simulink model "DFADAS2_SenFus_v1_201204RC_training_210115"  (R2018b)
settings: Solver=FixedStepDiscrete  StartTime=0.0  StopTime=inf  FixedStep=0.002  RelTol=1e-3  EnableMultiTasking=on
PreLoadFcn:
  | RTWConfigurationCB('preloadfcn', bdroot);
libraries: canmsglib x108, simulink x48, canfdmsglib x12
(part 28 of 28)

== system DFADAS2_SenFus_v1_201204RC_training_210115/Signal Input (Input)/Signal Input (50ms) (Input50)/Cmr/CmrInfo/L1 Information (L1Info)/CAN Diagnosis (CANDia)/CheckSum Diagnosis (ChkSumDia)/Bit Check(BChk)/Bit Operating (BOp)/ChksumPre4 ==
  In1 : Inport
  Data Type Conversion8 : DataTypeConversion  OutDataTypeStr=uint16
  Extract Bits1 : simulink/Logic and Bit Operations/Extract Bits  bitsToExtract=Range of bits  numBits=8  bitIdxRange=4  outScalingMode=Treat bit field as an integer
      settings: SourceProductName=Simulink
  Out1 : Outport
  wires:
  Extract Bits1/1 -> Data Type Conversion8/1
  In1/1 -> Extract Bits1/1
  Data Type Conversion8/1 -> Out1/1

== system DFADAS2_SenFus_v1_201204RC_training_210115/Signal Input (Input)/Signal Input (50ms) (Input50)/Cmr/CmrInfo/L1 Information (L1Info)/CAN Diagnosis (CANDia)/CheckSum Diagnosis (ChkSumDia)/Bit Check(BChk)/Bit Operating (BOp)/ChksumPre5 ==
  In1 : Inport
  In2 : Inport  Port=2
  Add : Sum
  Data Type Conversion1 : DataTypeConversion  OutDataTypeStr=uint16
  Data Type Conversion4 : DataTypeConversion  OutDataTypeStr=uint16
  Shift Arithmetic2 : ArithShift  BitShiftNumber=-8
  Out1 : Outport
  wires:
  In1/1 -> Data Type Conversion4/1
  In2/1 -> Data Type Conversion1/1
  Shift Arithmetic2/1 -> Add/1
  Add/1 -> Out1/1
  Data Type Conversion4/1 -> Shift Arithmetic2/1
  Data Type Conversion1/1 -> Add/2

== system DFADAS2_SenFus_v1_201204RC_training_210115/Signal Input (Input)/Signal Input (50ms) (Input50)/Cmr/CmrInfo/L1 Information (L1Info)/CAN Diagnosis (CANDia)/CheckSum Diagnosis (ChkSumDia)/Bit Check(BChk)/Bit Operating (BOp)/ChksumPre6 ==
  In1 : Inport
  In2 : Inport  Port=2
  Add : Sum
  Data Type Conversion1 : DataTypeConversion  OutDataTypeStr=uint16
  Data Type Conversion4 : DataTypeConversion  OutDataTypeStr=uint16
  Shift Arithmetic2 : ArithShift  BitShiftNumber=-8
  Out1 : Outport
  wires:
  Data Type Conversion1/1 -> Add/2
  Data Type Conversion4/1 -> Shift Arithmetic2/1
  Add/1 -> Out1/1
  Shift Arithmetic2/1 -> Add/1
  In2/1 -> Data Type Conversion1/1
  In1/1 -> Data Type Conversion4/1

== system DFADAS2_SenFus_v1_201204RC_training_210115/Signal Input (Input)/Signal Input (50ms) (Input50)/Cmr/CmrInfo/L1 Information (L1Info)/CAN Diagnosis (CANDia)/CheckSum Diagnosis (ChkSumDia)/Bit Check(BChk)/Bit Operating (BOp)/ChksumPre7 ==
  In1 : Inport
  Data Type Conversion8 : DataTypeConversion  OutDataTypeStr=uint16
  Extract Bits1 : simulink/Logic and Bit Operations/Extract Bits  bitsToExtract=Range of bits  numBits=8  bitIdxRange=7  outScalingMode=Treat bit field as an integer
      settings: SourceProductName=Simulink
  Out1 : Outport
  wires:
  Data Type Conversion8/1 -> Out1/1
  In1/1 -> Extract Bits1/1
  Extract Bits1/1 -> Data Type Conversion8/1

== system DFADAS2_SenFus_v1_201204RC_training_210115/Signal Input (Input)/Signal Input (50ms) (Input50)/Cmr/CmrInfo/R0 Information (R0Info)/CAN Diagnosis (CANDia)/CheckSum Diagnosis (ChkSumDia)/Bit Check(BChk)/Bit Operating (BOp)/ChksumPre1 ==
  In1 : Inport
  Data Type Conversion7 : DataTypeConversion  OutDataTypeStr=uint16
  Out1 : Outport
  wires:
  In1/1 -> Data Type Conversion7/1
  Data Type Conversion7/1 -> Out1/1

== system DFADAS2_SenFus_v1_201204RC_training_210115/Signal Input (Input)/Signal Input (50ms) (Input50)/Cmr/CmrInfo/R0 Information (R0Info)/CAN Diagnosis (CANDia)/CheckSum Diagnosis (ChkSumDia)/Bit Check(BChk)/Bit Operating (BOp)/ChksumPre2 ==
  In1 : Inport
  Data Type Conversion7 : DataTypeConversion  OutDataTypeStr=uint16
  Extract Bits : simulink/Logic and Bit Operations/Extract Bits  bitsToExtract=Range of bits  numBits=8  bitIdxRange=6  outScalingMode=Treat bit field as an integer
      settings: SourceProductName=Simulink
  Out1 : Outport
  wires:
  Data Type Conversion7/1 -> Out1/1
  In1/1 -> Extract Bits/1
  Extract Bits/1 -> Data Type Conversion7/1

== system DFADAS2_SenFus_v1_201204RC_training_210115/Signal Input (Input)/Signal Input (50ms) (Input50)/Cmr/CmrInfo/R0 Information (R0Info)/CAN Diagnosis (CANDia)/CheckSum Diagnosis (ChkSumDia)/Bit Check(BChk)/Bit Operating (BOp)/ChksumPre3 ==
  In1 : Inport
  Data Type Conversion8 : DataTypeConversion  OutDataTypeStr=uint16
  Extract Bits1 : simulink/Logic and Bit Operations/Extract Bits  bitsToExtract=Range of bits  numBits=8  bitIdxRange=5  outScalingMode=Treat bit field as an integer
      settings: SourceProductName=Simulink
  Out1 : Outport
  wires:
  Data Type Conversion8/1 -> Out1/1
  In1/1 -> Extract Bits1/1
  Extract Bits1/1 -> Data Type Conversion8/1

== system DFADAS2_SenFus_v1_201204RC_training_210115/Signal Input (Input)/Signal Input (50ms) (Input50)/Cmr/CmrInfo/R0 Information (R0Info)/CAN Diagnosis (CANDia)/CheckSum Diagnosis (ChkSumDia)/Bit Check(BChk)/Bit Operating (BOp)/ChksumPre4 ==
  In1 : Inport
  Data Type Conversion8 : DataTypeConversion  OutDataTypeStr=uint16
  Extract Bits1 : simulink/Logic and Bit Operations/Extract Bits  bitsToExtract=Range of bits  numBits=8  bitIdxRange=4  outScalingMode=Treat bit field as an integer
      settings: SourceProductName=Simulink
  Out1 : Outport
  wires:
  Extract Bits1/1 -> Data Type Conversion8/1
  In1/1 -> Extract Bits1/1
  Data Type Conversion8/1 -> Out1/1

== system DFADAS2_SenFus_v1_201204RC_training_210115/Signal Input (Input)/Signal Input (50ms) (Input50)/Cmr/CmrInfo/R0 Information (R0Info)/CAN Diagnosis (CANDia)/CheckSum Diagnosis (ChkSumDia)/Bit Check(BChk)/Bit Operating (BOp)/ChksumPre5 ==
  In1 : Inport
  In2 : Inport  Port=2
  Add : Sum
  Data Type Conversion1 : DataTypeConversion  OutDataTypeStr=uint16
  Data Type Conversion4 : DataTypeConversion  OutDataTypeStr=uint16
  Shift Arithmetic2 : ArithShift  BitShiftNumber=-8
  Out1 : Outport
  wires:
  In1/1 -> Data Type Conversion4/1
  In2/1 -> Data Type Conversion1/1
  Shift Arithmetic2/1 -> Add/1
  Add/1 -> Out1/1
  Data Type Conversion4/1 -> Shift Arithmetic2/1
  Data Type Conversion1/1 -> Add/2

== system DFADAS2_SenFus_v1_201204RC_training_210115/Signal Input (Input)/Signal Input (50ms) (Input50)/Cmr/CmrInfo/R0 Information (R0Info)/CAN Diagnosis (CANDia)/CheckSum Diagnosis (ChkSumDia)/Bit Check(BChk)/Bit Operating (BOp)/ChksumPre6 ==
  In1 : Inport
  In2 : Inport  Port=2
  Add : Sum
  Data Type Conversion1 : DataTypeConversion  OutDataTypeStr=uint16
  Data Type Conversion4 : DataTypeConversion  OutDataTypeStr=uint16
  Shift Arithmetic2 : ArithShift  BitShiftNumber=-8
  Out1 : Outport
  wires:
  Data Type Conversion1/1 -> Add/2
  Data Type Conversion4/1 -> Shift Arithmetic2/1
  Add/1 -> Out1/1
  Shift Arithmetic2/1 -> Add/1
  In2/1 -> Data Type Conversion1/1
  In1/1 -> Data Type Conversion4/1

== system DFADAS2_SenFus_v1_201204RC_training_210115/Signal Input (Input)/Signal Input (50ms) (Input50)/Cmr/CmrInfo/R0 Information (R0Info)/CAN Diagnosis (CANDia)/CheckSum Diagnosis (ChkSumDia)/Bit Check(BChk)/Bit Operating (BOp)/ChksumPre7 ==
  In1 : Inport
  Data Type Conversion8 : DataTypeConversion  OutDataTypeStr=uint16
  Extract Bits1 : simulink/Logic and Bit Operations/Extract Bits  bitsToExtract=Range of bits  numBits=8  bitIdxRange=7  outScalingMode=Treat bit field as an integer
      settings: SourceProductName=Simulink
  Out1 : Outport
  wires:
  Data Type Conversion8/1 -> Out1/1
  In1/1 -> Extract Bits1/1
  Extract Bits1/1 -> Data Type Conversion8/1

== system DFADAS2_SenFus_v1_201204RC_training_210115/Signal Input (Input)/Signal Input (50ms) (Input50)/Cmr/CmrInfo/R1 Information (R1Info)/CAN Diagnosis (CANDia)/CheckSum Diagnosis (ChkSumDia)/Bit Check(BChk)/Bit Operating (BOp)/ChksumPre1 ==
  In1 : Inport
  Data Type Conversion7 : DataTypeConversion  OutDataTypeStr=uint16
  Out1 : Outport
  wires:
  Data Type Conversion7/1 -> Out1/1
  In1/1 -> Data Type Conversion7/1

== system DFADAS2_SenFus_v1_201204RC_training_210115/Signal Input (Input)/Signal Input (50ms) (Input50)/Cmr/CmrInfo/R1 Information (R1Info)/CAN Diagnosis (CANDia)/CheckSum Diagnosis (ChkSumDia)/Bit Check(BChk)/Bit Operating (BOp)/ChksumPre2 ==
  In1 : Inport
  Data Type Conversion7 : DataTypeConversion  OutDataTypeStr=uint16
  Extract Bits : simulink/Logic and Bit Operations/Extract Bits  bitsToExtract=Range of bits  numBits=8  bitIdxRange=6  outScalingMode=Treat bit field as an integer
      settings: SourceProductName=Simulink
  Out1 : Outport
  wires:
  Extract Bits/1 -> Data Type Conversion7/1
  In1/1 -> Extract Bits/1
  Data Type Conversion7/1 -> Out1/1

== system DFADAS2_SenFus_v1_201204RC_training_210115/Signal Input (Input)/Signal Input (50ms) (Input50)/Cmr/CmrInfo/R1 Information (R1Info)/CAN Diagnosis (CANDia)/CheckSum Diagnosis (ChkSumDia)/Bit Check(BChk)/Bit Operating (BOp)/ChksumPre3 ==
  In1 : Inport
  Data Type Conversion8 : DataTypeConversion  OutDataTypeStr=uint16
  Extract Bits1 : simulink/Logic and Bit Operations/Extract Bits  bitsToExtract=Range of bits  numBits=8  bitIdxRange=5  outScalingMode=Treat bit field as an integer
      settings: SourceProductName=Simulink
  Out1 : Outport
  wires:
  Extract Bits1/1 -> Data Type Conversion8/1
  In1/1 -> Extract Bits1/1
  Data Type Conversion8/1 -> Out1/1

== system DFADAS2_SenFus_v1_201204RC_training_210115/Signal Input (Input)/Signal Input (50ms) (Input50)/Cmr/CmrInfo/R1 Information (R1Info)/CAN Diagnosis (CANDia)/CheckSum Diagnosis (ChkSumDia)/Bit Check(BChk)/Bit Operating (BOp)/ChksumPre4 ==
  In1 : Inport
  Data Type Conversion8 : DataTypeConversion  OutDataTypeStr=uint16
  Extract Bits1 : simulink/Logic and Bit Operations/Extract Bits  bitsToExtract=Range of bits  numBits=8  bitIdxRange=4  outScalingMode=Treat bit field as an integer
      settings: SourceProductName=Simulink
  Out1 : Outport
  wires:
  Data Type Conversion8/1 -> Out1/1
  In1/1 -> Extract Bits1/1
  Extract Bits1/1 -> Data Type Conversion8/1

== system DFADAS2_SenFus_v1_201204RC_training_210115/Signal Input (Input)/Signal Input (50ms) (Input50)/Cmr/CmrInfo/R1 Information (R1Info)/CAN Diagnosis (CANDia)/CheckSum Diagnosis (ChkSumDia)/Bit Check(BChk)/Bit Operating (BOp)/ChksumPre5 ==
  In1 : Inport
  In2 : Inport  Port=2
  Add : Sum
  Data Type Conversion1 : DataTypeConversion  OutDataTypeStr=uint16
  Data Type Conversion4 : DataTypeConversion  OutDataTypeStr=uint16
  Shift Arithmetic2 : ArithShift  BitShiftNumber=-8
  Out1 : Outport
  wires:
  Data Type Conversion1/1 -> Add/2
  Data Type Conversion4/1 -> Shift Arithmetic2/1
  Add/1 -> Out1/1
  Shift Arithmetic2/1 -> Add/1
  In2/1 -> Data Type Conversion1/1
  In1/1 -> Data Type Conversion4/1

== system DFADAS2_SenFus_v1_201204RC_training_210115/Signal Input (Input)/Signal Input (50ms) (Input50)/Cmr/CmrInfo/R1 Information (R1Info)/CAN Diagnosis (CANDia)/CheckSum Diagnosis (ChkSumDia)/Bit Check(BChk)/Bit Operating (BOp)/ChksumPre6 ==
  In1 : Inport
  In2 : Inport  Port=2
  Add : Sum
  Data Type Conversion1 : DataTypeConversion  OutDataTypeStr=uint16
  Data Type Conversion4 : DataTypeConversion  OutDataTypeStr=uint16
  Shift Arithmetic2 : ArithShift  BitShiftNumber=-8
  Out1 : Outport
  wires:
  In1/1 -> Data Type Conversion4/1
  In2/1 -> Data Type Conversion1/1
  Shift Arithmetic2/1 -> Add/1
  Add/1 -> Out1/1
  Data Type Conversion4/1 -> Shift Arithmetic2/1
  Data Type Conversion1/1 -> Add/2

== system DFADAS2_SenFus_v1_201204RC_training_210115/Signal Input (Input)/Signal Input (50ms) (Input50)/Cmr/CmrInfo/R1 Information (R1Info)/CAN Diagnosis (CANDia)/CheckSum Diagnosis (ChkSumDia)/Bit Check(BChk)/Bit Operating (BOp)/ChksumPre7 ==
  In1 : Inport
  Data Type Conversion8 : DataTypeConversion  OutDataTypeStr=uint16
  Extract Bits1 : simulink/Logic and Bit Operations/Extract Bits  bitsToExtract=Range of bits  numBits=8  bitIdxRange=7  outScalingMode=Treat bit field as an integer
      settings: SourceProductName=Simulink
  Out1 : Outport
  wires:
  Extract Bits1/1 -> Data Type Conversion8/1
  In1/1 -> Extract Bits1/1
  Data Type Conversion8/1 -> Out1/1
